simulink model "fluxrampdemodulationb"  (R2012b)
settings: Solver=ode45  StartTime=0.0  StopTime=10000  RelTol=1e-3
undefined symbols (not defined in the file): SL, transtable
libraries: xbsIndex_r4 x1338, casper_library_misc x8, xps_library x1
(part 1 of 13)
settings Model: Creator=tmadden  LastModifiedBy=tmadden

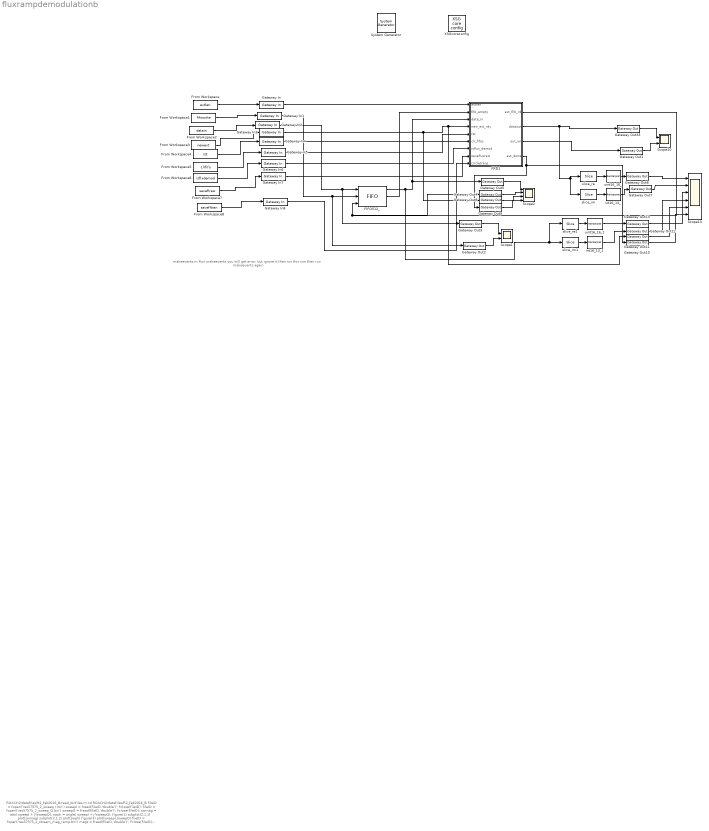
== system fluxrampdemodulationb ==
  note: makeevents.m
      | Run makeevents
      | you will get error, but ignore it
      | then run this sim
      | then run makeevents again
  note: ROACH2/datefiles/R2_feb2016_B/read_binfiles.m
      | cd ROACH2/datefiles/R2_feb2016_B
      |
      |
      |
      |
      |
      | fileID = fopen('res57575_2_sweep_I.bin')
      | sweepI = fread(fileID,'double')';
      | fclose(fileID);
      |
      |
      | fileID = fopen('res57575_2_sweep_Q.bin')
      | sweepQ = fread(fileID,'double')';
      | fclose(fileID);
      |
      |
      | swmag = abs( sweepI + j*sweepQ);
      |
      | swph = angle( sweepI + j*sweepQ);
      |
      | figure(1)
      | subplot(2,1,1)
      | plot(swmag)
      | subplot(2,1,2)
      | plot(swph)
      |
      | figure(3)
      | plot(sweepI,sweepQ)
      |
      |
      | fileID = fopen('res57575_2_stream_mag_ramp.bin')
      | mags = fread(fileID,'double')';
      | fclose(fileID);
      |
      |
      | fileID = fopen('res_57575_2_stream_phase_ramp.bin')
      | phasesr = fread(fileID,'double')';
      | fclose(fileID);
      |
      |
      |
      | nI = mags .* cos(phasesr);
      | nQ = mags .* sin(phasesr);
      |
      |
      | figure(3)
      | hold on
      | plot(nI,nQ,'r.')
      |
      |
      |
      |
      |
      | phases = phasesr / (pi);
      | phases = phases - 346;
      |
      |
      |
      | phases = [swph/pi , phases];
      | figure(4)
      | plot(phases(1:1000))
      |
      |
      | mags = [swmag , mags];
      |
      | magtime = timeseries(mags);
      | phasetime = timeseries(phases);
      |
      |
      | sync = zeros(1,length(phases));
      |
      | ping = 350;
      |
      | i = ping:100:length(phases);
      | sync(i) = 1;
      |
      |
      | synctime = timeseries(sync)
      |
      | figure(4)
      |
      | subplot(3,1,1)
      | plot(mags(1:400))
      | subplot(3,1,2)
      | plot(phases(1:400))
      | subplot(3,1,3)
      | plot(sync(1:400))
  " System Generator" : xbsIndex_r4/ System Generator  Tag=genX  xilinxfamily=Kintex7  part=xc7k325t  speed=-3  package=fbg676  synthesis_tool=XST  clock_wrapper=Clock Enables  directory=./netlist  proj_type=Project Navigator  Synth_file=XST Defaults  Impl_file=ISE Defaults  testbench=off  simulink_period=1  sysclk_period=10  dcm_input_clock_period=10  incr_netlist=off  trim_vbits=Everywhere in SubSystem  dbl_ovrd=According to Block Masks  core_generation=According to Block Masks  run_coregen=off  deprecated_control=off  eval_field=0  block_type=sysgen
  FIFO512_ : xbsIndex_r4/FIFO  mem_type=Block RAM  performance_options=First_Word_Fall_Through  infoedit1=Available only for V4, V5, V6, V7, K7, A7 and Zynq devices.  embedded_registers=off  depth=512  percent_nbits=1  rst=off  en=off  use_dcount=off  use_percent_full_port=off  use_almost_empty=off  almost_empty_thresh=2  use_almost_full=off  almost_full_thresh=256  dbl_ovrd=off  explicit_period=off  block_type=fifo
  FRD1 : Subsystem
  From Workspace : FromWorkspace  VariableName=evtlen  SampleTime=0  OutputAfterFinalValue=Holding final value
  From Workspace1 : FromWorkspace  VariableName=fifowrite  SampleTime=0  OutputAfterFinalValue=Holding final value
  From Workspace2 : FromWorkspace  VariableName=datain  Interpolate=off  OutputAfterFinalValue=Holding final value
  From Workspace3 : FromWorkspace  VariableName=newevt  SampleTime=0  OutputAfterFinalValue=Holding final value
  From Workspace4 : FromWorkspace  VariableName=rst  SampleTime=0  OutputAfterFinalValue=Holding final value
  From Workspace5 : FromWorkspace  VariableName=clrfifo  SampleTime=0  OutputAfterFinalValue=Holding final value
  From Workspace6 : FromWorkspace  VariableName=isflxdemod  SampleTime=0  OutputAfterFinalValue=Holding final value
  From Workspace7 : FromWorkspace  VariableName=saveflraw  SampleTime=0  OutputAfterFinalValue=Holding final value
  From Workspace8 : FromWorkspace  VariableName=savefltran  SampleTime=0  OutputAfterFinalValue=Holding final value
  Gateway In : xbsIndex_r4/Gateway In  gui_display_data_type=Fixed-point  arith_type=Unsigned  n_bits=8  bin_pt=0  preci_type=Single  exp_width=8  frac_width=24  quantization="Round  (unbiased: +/- Inf)"  overflow=Saturate  period=1  dbl_ovrd=off  timing_constraint=None  locs_specified=off  LOCs={}  UseAsADC=off  ADCChannel='1'  inherit_from_input=off  hdl_port=on  block_type=gatewayin
  Gateway In{1,3..8} (7 alike) : xbsIndex_r4/Gateway In  gui_display_data_type=Boolean  arith_type=Boolean  n_bits=16  bin_pt=14  preci_type=Single  exp_width=8  frac_width=24  quantization="Round  (unbiased: +/- Inf)"  overflow=Saturate  period=1  dbl_ovrd=off  timing_constraint=None  locs_specified=off  LOCs={}  UseAsADC=off  ADCChannel='1'  inherit_from_input=off  hdl_port=on  block_type=gatewayin
  Gateway In2 : xbsIndex_r4/Gateway In  gui_display_data_type=Fixed-point  arith_type=Unsigned  n_bits=32  bin_pt=0  preci_type=Single  exp_width=8  frac_width=24  quantization="Round  (unbiased: +/- Inf)"  overflow=Saturate  period=1  dbl_ovrd=off  timing_constraint=None  locs_specified=off  LOCs={}  UseAsADC=off  ADCChannel='1'  inherit_from_input=off  hdl_port=on  block_type=gatewayin
  Gateway Out{1..13,33} (14 alike) : xbsIndex_r4/Gateway Out  inherit_from_input=off  hdl_port=on  timing_constraint=None  locs_specified=off  LOCs={}  UseAsDAC=off  DACChannel='1'  block_type=gatewayout
  Scope1 : Scope  NumInputPorts=2
      settings: YMin=-5~-5  YMax=5~5  SaveName=output1  MaxDataPoints=1800
  Scope10 : Scope  NumInputPorts=2
      settings: YMin=-5~-5  YMax=5~5  SaveName=output  MaxDataPoints=1800
  Scope13 : Scope  NumInputPorts=6
      settings: YMin=-5~-5~-5~-5~-5~-5  YMax=5~5~5~5~5~5  SaveName=output3  MaxDataPoints=1800
  Scope2 : Scope  NumInputPorts=4
      settings: YMin=-5~-5~-5~-5  YMax=5~5~5~5  SaveName=output2  MaxDataPoints=1800
  XSGcoreconfig : xps_library/XSG core config  Tag=xps:xsg  hw_sys=ROACH2:sx475t  clk_src=sys_clk  ROACH_clk_src=sys_clk  ROACH2_clk_src=sys_clk  MKDIG_clk_src=sys_clk  clk_rate=128  sample_period=1  synthesis_tool=XST
  int16_13_ : xbsIndex_r4/Reinterpret  force_arith_type=on  arith_type="Signed  (2's comp)"  force_bin_pt=on  bin_pt=13  block_type=reinterpret
      settings: block_version=9.1.01
  int16_13_1 : xbsIndex_r4/Reinterpret  force_arith_type=on  arith_type="Signed  (2's comp)"  force_bin_pt=on  bin_pt=13  block_type=reinterpret
      settings: block_version=9.1.01
  slice_im : xbsIndex_r4/Slice  nbits=16  boolean_output=off  mode=Lower Bit Location + Width  bit1=0  base1=MSB of Input  bit0=0  base0=LSB of Input  dbl_ovrd=off  block_type=slice
      settings: block_version=9.1.01
  slice_im1 : xbsIndex_r4/Slice  nbits=16  boolean_output=off  mode=Lower Bit Location + Width  bit1=0  base1=MSB of Input  bit0=0  base0=LSB of Input  dbl_ovrd=off  block_type=slice
      settings: block_version=9.1.01
  slice_re : xbsIndex_r4/Slice  nbits=16  boolean_output=off  mode=Upper Bit Location + Width  bit1=0  base1=MSB of Input  bit0=0  base0=LSB of Input  dbl_ovrd=off  block_type=slice
      settings: block_version=9.1.01
  slice_re1 : xbsIndex_r4/Slice  nbits=16  boolean_output=off  mode=Upper Bit Location + Width  bit1=0  base1=MSB of Input  bit0=0  base0=LSB of Input  dbl_ovrd=off  block_type=slice
      settings: block_version=9.1.01
  uint16_16_ : xbsIndex_r4/Reinterpret  force_arith_type=on  arith_type=Unsigned  force_bin_pt=on  bin_pt=16  block_type=reinterpret
      settings: block_version=9.1.01
  uint16_16_1 : xbsIndex_r4/Reinterpret  force_arith_type=on  arith_type=Unsigned  force_bin_pt=on  bin_pt=16  block_type=reinterpret
      settings: block_version=9.1.01
  wires:
  Gateway In/1 -> FRD1/1(evtlen)
  Gateway In4/1 -> FRD1/5(rst)
  Gateway In5/1 -> FRD1/6(clr_fifos)
  Gateway In6/1 -> FRD1/7(isflux_demod)
  Gateway In7/1 -> FRD1/8(savefluxraw)
  From Workspace/1 -> Gateway In/1
  From Workspace1/1 -> Gateway In1/1
  From Workspace2/1 -> Gateway In2/1
  From Workspace3/1 -> Gateway In3/1
  From Workspace4/1 -> Gateway In4/1
  From Workspace5/1 -> Gateway In5/1
  From Workspace6/1 -> Gateway In6/1
  From Workspace7/1 -> Gateway In7/1
  Gateway Out33/1 -> Scope10/1
  FRD1/2(dataout) -> slice_im/1, slice_re/1, Gateway Out33/1
  Gateway Out1/1 -> Scope10/2
  FRD1/3(out_wr) -> Gateway Out1/1
  Gateway Out3/1 -> Scope1/1
  Gateway Out2/1 -> Scope1/2
  Gateway In3/1 -> Gateway Out8/1, FRD1/4(new_evt_rdy), Gateway Out11/1
  Gateway In2/1 -> Gateway Out3/1, FIFO512_/1
  FIFO512_/1 -> slice_re1/1, slice_im1/1, FRD1/3(data_in), Gateway Out5/1
  FRD1/1(evt_fifo_rd) -> FIFO512_/3, Gateway Out4/1
  FIFO512_/2 -> FRD1/2(fifo_empty)
  Gateway In1/1 -> Gateway Out2/1, FIFO512_/2
  Gateway Out5/1 -> Scope2/1
  Gateway Out4/1 -> Scope2/2
  From Workspace8/1 -> Gateway In8/1
  Gateway In8/1 -> FRD1/9(circletrans)
  slice_re/1 -> uint16_16_/1
  slice_im/1 -> int16_13_/1
  uint16_16_/1 -> Gateway Out6/1
  Gateway Out6/1 -> Scope13/1
  int16_13_/1 -> Gateway Out7/1
  Gateway Out7/1 -> Scope13/2
  Gateway Out8/1 -> Scope2/3
  Gateway Out9/1 -> Scope2/4
  FRD1/4(evt_done) -> Gateway Out10/1, Gateway Out9/1
  slice_re1/1 -> uint16_16_1/1
  slice_im1/1 -> int16_13_1/1
  uint16_16_1/1 -> Gateway Out13/1
  int16_13_1/1 -> Gateway Out12/1
  Gateway Out13/1 -> Scope13/3
  Gateway Out12/1 -> Scope13/4
  Gateway Out11/1 -> Scope13/5
  Gateway Out10/1 -> Scope13/6

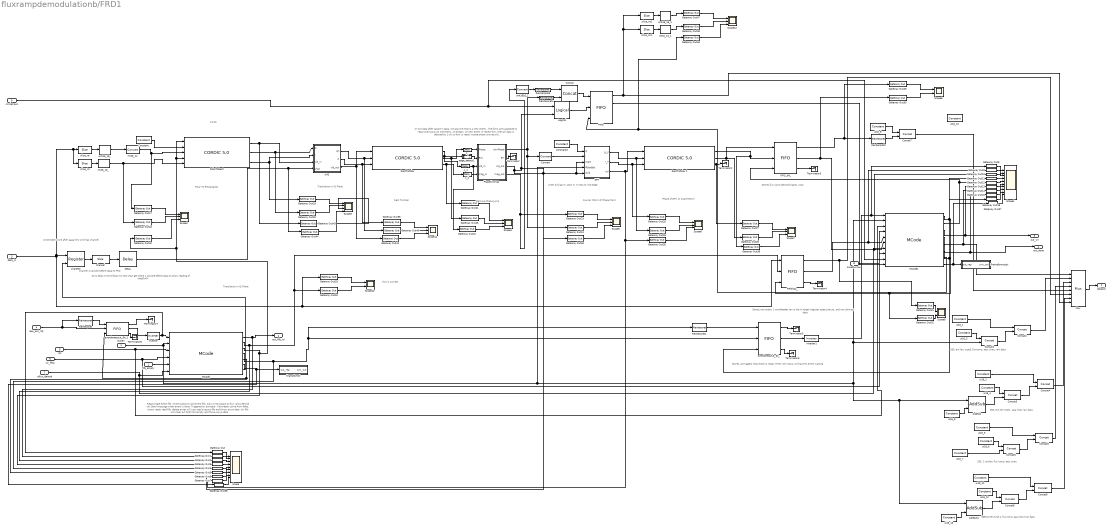
== system fluxrampdemodulationb/FRD1 ==
  note: stroe 32bit word after aaaa
      | this wird has channel
  note: 20 is delay time of polar to rect
      | chan get there 1 sample before data
      | to allow reading of theBRAM
  note: channel 1 sample before
      | data to FRD
  note: Z=20
  note: on 1st data after pause in data, we assume that is a new event...
      | the fsms are supposed to read continuous on one event...no breaks.
      | on new event, it resets fsm. then all data is delayed bu 1 clk so fsm
      | is ready insode phase unwrap ckt.
  note: this is correct
  note: 555, evt len type1 , aaa chan raw data
  note: 555, evt len, type3, fluxramp, aaa, chan, raw data
  note: 555, 2, evtlen, flux ramp, aaa, chan,
  note: Stores flux ramp dempd [hases. chan
  note: when dvld go hi, start it. it resp to rise edge
  note: Polar To Rectangular
  note: Translation in IQ Plane
  note: Remove Phase Jump
  note: Fourier Xform
      | Of Phase Term
  note: Rect To Polar
  note: Phase of DFT,
      | or Atan(Re/Im)
  note: Translation in IQ Plane
  note: Stores raw event.
      | 2 wordheader
      | len is the in length register
      | aaaa,chan,ts, and raw ph/mag data
  note: Stores up triggers that event is ready
      | When not mptuy we have en event waiting
  note: Read single event fifo.
      | Write output to 2nd event fifo.
      | Also write output to flux ramp demod ckt
      | Send message when event is done.
      | Triggered by evtready. if evtready come from fofop, clrevt ready read fifo.
      | delete evnet will just read sing evt fifo and throw awya data.
      | ckr fifo will clear evt fuifo intil empty and throw awya data
  note: 5555,evlen,type 4, fluxramp, aaa chan tran data
  evtlen : Inport
  fifo_empty : Inport  Port=2
  data_in : Inport  Port=3
  new_evt_rdy : Inport  Port=4
  rst : Inport  Port=5
  clr_fifos : Inport  Port=6
  isflux_demod : Inport  Port=7
  savefluxraw : Inport  Port=8
  circletrans : Inport  Port=9
  AddSub : xbsIndex_r4/AddSub  mode=Addition  use_carryin=off  use_carryout=off  en=off  latency=1  precision=User Defined  arith_type=Unsigned  n_bits=8  bin_pt=0  quantization=Truncate  overflow=Wrap  dbl_ovrd=off  use_behavioral_HDL=off  hw_selection=Fabric  pipelined=off  block_type=addsub
  AddSub1 : xbsIndex_r4/AddSub  mode=Addition  use_carryin=off  use_carryout=off  en=off  latency=1  precision=User Defined  arith_type=Unsigned  n_bits=8  bin_pt=0  quantization=Truncate  overflow=Wrap  dbl_ovrd=off  use_behavioral_HDL=off  hw_selection=Fabric  pipelined=off  block_type=addsub
  Concat{,1..9} (10 alike) : xbsIndex_r4/Concat  num_inputs=2  dbl_ovrd=off  block_type=concat
  Constant : xbsIndex_r4/Constant  const=0  gui_display_data_type=Fixed-point  arith_type=Signed (2's comp)  n_bits=16  bin_pt=14  preci_type=Single  exp_width=8  frac_width=24  explicit_period=on  period=1  equ=P=C  opselect=C  inp2=PCIN>>17  opr=+  inp1=P  carry=CIN  dbl_ovrd=off  block_type=constant
  Constant3 : xbsIndex_r4/Constant  const=0  gui_display_data_type=Fixed-point  arith_type=Signed (2's comp)  n_bits=16  bin_pt=14  preci_type=Single  exp_width=8  frac_width=24  explicit_period=on  period=1  equ=P=C  opselect=C  inp2=PCIN>>17  opr=+  inp1=P  carry=CIN  dbl_ovrd=off  block_type=constant
  Convert : xbsIndex_r4/Convert  gui_display_data_type=Fixed-point  arith_type="Signed  (2's comp)"  n_bits=16  bin_pt=14  float_type=Single  exp_bits=8  fraction_bits=24  quantization=Truncate  overflow=Wrap  en=off  latency=0  dbl_ovrd=off  pipeline=off  block_type=convert
  DFT : Subsystem
  Delay : xbsIndex_r4/Delay  rst=off  infoeditControl=Selection of Reset will increase slice count due to use of real FFs and instead of SRLs  en=off  latency=19  dbl_ovrd=off  reg_retiming=off  block_type=delay
  FIFO : xbsIndex_r4/FIFO  mem_type=Block RAM  performance_options=First_Word_Fall_Through  infoedit1=Available only for V4, V5, V6, V7, K7, A7 and Zynq devices.  embedded_registers=off  depth=512  percent_nbits=1  rst=off  en=off  use_dcount=off  use_percent_full_port=on  use_almost_empty=off  almost_empty_thresh=2  use_almost_full=off  almost_full_thresh=14  dbl_ovrd=off  explicit_period=off  block_type=fifo
  FIFO512_ : xbsIndex_r4/FIFO  mem_type=Block RAM  performance_options=First_Word_Fall_Through  infoedit1=Available only for V4, V5, V6, V7, K7, A7 and Zynq devices.  embedded_registers=off  depth=512  percent_nbits=1  rst=off  en=off  use_dcount=off  use_percent_full_port=off  use_almost_empty=off  almost_empty_thresh=2  use_almost_full=off  almost_full_thresh=256  dbl_ovrd=off  explicit_period=off  block_type=fifo
  FIFO_64_ : xbsIndex_r4/FIFO  mem_type=Block RAM  performance_options=First_Word_Fall_Through  infoedit1=Available only for V4, V5, V6, V7, K7, A7 and Zynq devices.  embedded_registers=off  depth=64  percent_nbits=1  rst=off  en=off  use_dcount=off  use_percent_full_port=off  use_almost_empty=off  almost_empty_thresh=2  use_almost_full=off  almost_full_thresh=32  dbl_ovrd=off  explicit_period=off  block_type=fifo
  Gateway Out{,1..49} (50 alike) : xbsIndex_r4/Gateway Out  inherit_from_input=off  hdl_port=on  timing_constraint=None  locs_specified=off  LOCs={}  UseAsDAC=off  DACChannel='1'  block_type=gatewayout
  Inverter : xbsIndex_r4/Inverter  en=off  latency=0  dbl_ovrd=off  block_type=inv
  Inverter1 : xbsIndex_r4/Inverter  en=off  latency=0  dbl_ovrd=off  block_type=inv
  Logical : xbsIndex_r4/Logical  logical_function=AND  inputs=2  en=off  latency=0  precision=Full  arith_type=Unsigned  n_bits=16  bin_pt=0  align_bp=on  dbl_ovrd=off  block_type=logical
  MCode : xbsIndex_r4/MCode  mfname=fluxRampFSM.m  explicit_period=off  period=1  inputsTable={'boundInpExpr'=>['','','','','',''],'inputs'=>['event_rdy','event_length','rst','clr_fifos','fifo_empty','is_fluxrampdemod']}  outputsTable={'outputs'=>['eventfifo_rd','outfifo_wr','demod_wr','event_done','clr_evt_rdy','stout'],'suppressOut'=>['off','off','off','off','off','off']}  dbl_ovrd=off  enable_stdout=off  enable_debug=off  suppress_output=on  defparams={}  hide_port_list={}  block_type=mcode
  MCode1 : xbsIndex_r4/MCode  mfname=fluxRampFSMOut2  explicit_period=on  period=1  inputsTable={'boundInpExpr'=>['','','','','','','',''],'inputs'=>['event_rdy','event_length','rst','clr_fifos','rawevt_fifo_empty','fluxrmp_fifo_empy','is_fluxrampdemod','is_savefluxraw']}  outputsTable={'outputs'=>['eventfifo_rd','fluxfifo_rd','outfifo_wr','wr_select','event_done','clr_evt_rdy','stout'],'suppressOut'=>['off','off','off','off','off','off','off']}  dbl_ovrd=off  enable_stdout=off  enable_debug=off  suppress_output=on  defparams={}  hide_port_list={}  block_type=mcode
  Mux : xbsIndex_r4/Mux  inputs=7  en=off  latency=0  precision=Full  arith_type=Unsigned  n_bits=16  bin_pt=14  quantization=Truncate  overflow=Wrap  dbl_ovrd=off  block_type=mux
  PhaseUnwrap : Subsystem
  "PolarToRect " : xbsIndex_r4/CORDIC 5.0   functional_selection=Rotate  architectural_configuration=Parallel  pipelining_mode=Maximum  data_format=SignedFraction  phase_format=Scaled_Radians  input_width=16  output_width=16  round_mode=Truncate  iterations=0  precision=0  compensation_scaling=Embedded_Multiplier  coarse_rotation=on  aclken=off  aresetn=off  out_tready=off  cartesian_has_tuser=off  cartesian_has_tlast=off  cartesian_tuser_width=1  phase_has_tuser=off  phase_has_tlast=off  phase_tuser_width=1  out_tlast_behv=Null  flow_control=NonBlocking  optimize_goal=Performance  trim_axipin_name=on  ip_name=CORDIC  ip_version=5.0  dsptool_ready=true  ipcore_usecache=true  ipcore_useipmodelcache=true  wrapper_available=true  port_translation_map={ 'aclken' => 'en', 'aresetn' => 'rst' }  block_type=cordic_v5_0
      settings: infoedit=CORDIC 5.0
  "RectToPolar " : xbsIndex_r4/CORDIC 5.0   functional_selection=Translate  architectural_configuration=Parallel  pipelining_mode=Maximum  data_format=SignedFraction  phase_format=Scaled_Radians  input_width=16  output_width=16  round_mode=Truncate  iterations=0  precision=0  compensation_scaling=Embedded_Multiplier  coarse_rotation=on  aclken=off  aresetn=off  out_tready=off  cartesian_has_tuser=off  cartesian_has_tlast=off  cartesian_tuser_width=1  phase_has_tuser=off  phase_has_tlast=off  phase_tuser_width=1  out_tlast_behv=Null  flow_control=NonBlocking  optimize_goal=Performance  trim_axipin_name=on  ip_name=CORDIC  ip_version=5.0  dsptool_ready=true  ipcore_usecache=true  ipcore_useipmodelcache=true  wrapper_available=true  port_translation_map={ 'aclken' => 'en', 'aresetn' => 'rst' }  block_type=cordic_v5_0
      settings: infoedit=CORDIC 5.0
  RectToPolar 1 : xbsIndex_r4/CORDIC 5.0   functional_selection=Translate  architectural_configuration=Parallel  pipelining_mode=Maximum  data_format=SignedFraction  phase_format=Scaled_Radians  input_width=16  output_width=16  round_mode=Truncate  iterations=0  precision=0  compensation_scaling=Embedded_Multiplier  coarse_rotation=on  aclken=off  aresetn=off  out_tready=off  cartesian_has_tuser=off  cartesian_has_tlast=off  cartesian_tuser_width=1  phase_has_tuser=off  phase_has_tlast=off  phase_tuser_width=1  out_tlast_behv=Null  flow_control=NonBlocking  optimize_goal=Performance  trim_axipin_name=on  ip_name=CORDIC  ip_version=5.0  dsptool_ready=true  ipcore_usecache=true  ipcore_useipmodelcache=true  wrapper_available=true  port_translation_map={ 'aclken' => 'en', 'aresetn' => 'rst' }  block_type=cordic_v5_0
      settings: infoedit=CORDIC 5.0
  Reinterpret : xbsIndex_r4/Reinterpret  force_arith_type=on  arith_type=Unsigned  force_bin_pt=off  bin_pt=0  block_type=reinterpret
  Reinterpret1 : xbsIndex_r4/Reinterpret  force_arith_type=on  arith_type=Unsigned  force_bin_pt=off  bin_pt=0  block_type=reinterpret
  Reinterpret2 : xbsIndex_r4/Reinterpret  force_arith_type=on  arith_type=Unsigned  force_bin_pt=on  bin_pt=0  block_type=reinterpret
  Reinterpret3 : xbsIndex_r4/Reinterpret  force_arith_type=on  arith_type=Unsigned  force_bin_pt=on  bin_pt=0  block_type=reinterpret
  Reinterpret4 : xbsIndex_r4/Reinterpret  force_arith_type=on  arith_type=Unsigned  force_bin_pt=on  bin_pt=0  block_type=reinterpret
  Scope : Scope  NumInputPorts=9
      settings: YMin=-5~-5~-5~-5~-5~-5~-5~-5~-5  YMax=5~5~5~5~5~5~5~5~5  SaveName=boolscope2
  Scope1 : Scope  NumInputPorts=10
      settings: YMin=-5~-5~-5~-5~-5~-5~-5~-5~-5~-5  YMax=5~5~5~5~5~5~5~5~5~5  SaveName=boolscope3
  Scope10 : Scope  NumInputPorts=2
      settings: YMin=-5~-5  YMax=5~5  SaveName=outfsm2  MaxDataPoints=1800
  Scope{2,4..7,11..12} (7 alike) : Scope  NumInputPorts=3
      Scope11 settings: TimeRange=1240.478781284003  YMin=-5~-5~-5  YMax=5~5~5  SaveName=scope_aftertr  MaxDataPoints=1800
      Scope12 settings: YMin=-5~-5~-5  YMax=5~5~5  SaveName=ScopeData18  MaxDataPoints=1800
      Scope2 settings: YMin=-5~-5~-5  YMax=5~5~5  MaxDataPoints=1800
      Scope4 settings: YMin=-5~-5~-5  YMax=5~5~5  SaveName=ScopeData3  MaxDataPoints=1800
      Scope5 settings: YMin=-5~-5~-5  YMax=5~5~5  SaveName=ScopeData4  MaxDataPoints=1800
      Scope6 settings: YMin=-5~-5~-5  YMax=5~5~5  SaveName=ScopeData6  MaxDataPoints=1800
      Scope7 settings: YMin=-5~-5~-5  YMax=5~5~5  SaveName=outdftdata  MaxDataPoints=1800
  Scope3 : Scope  NumInputPorts=4
      settings: TimeRange=1240.478781284003  YMin=-5~-5~-5~-5  YMax=5~5~5~5  SaveName=scope_beforetr  MaxDataPoints=1800
  Scope8 : Scope  NumInputPorts=2
      settings: YMin=-5~-5  YMax=5~5  SaveName=ScopeData15  MaxDataPoints=1800
  Scope9 : Scope  NumInputPorts=2
      settings: YMin=-5~-5  YMax=5~5  SaveName=ScopeData16  MaxDataPoints=1800
  Terminator{,2..8} (8 alike) : Terminator
  chanReg : xbsIndex_r4/Register  init=0  rst=off  en=on  dbl_ovrd=off  block_type=register
  channel : xbsIndex_r4/Slice  nbits=8  boolean_output=off  mode=Lower Bit Location + Width  bit1=0  base1=MSB of Input  bit0=0  base0=LSB of Input  dbl_ovrd=off  block_type=slice
  edge_detect1 : Subsystem  AncestorBlock=casper_library_misc/edge_detect  mask(edge_detect){edge=Rising, polarity=Active High, x_in=[0 0.08 0.08 0.16 0.16 0.24 0.24 0.32 0.32 0.4], y_in=[-1 -1  1  1  1  1  1  1  1  1], x_out=[0.6 0.68 0.68 0.76 0.76 0.84 0.84 0.92 0.92 1], y_out=[-1 -1  1  1 -1 -1 -1 -1 -1 -1]}
      mask prompts: edge "Edge Type"; polarity "Output Polarity"; x_in "Input X Positions"; y_in "Input Y Positions"; x_out "Output X Positions"; y_out "Output Y Positions"
      mask help: Output is active for one-cycle after each edge of the specified type (i.e. rising, falling or both).
      mask init:
      | edge_detect_init(gcb,...
      |     'edge',edge,...
      |     'polarity',polarity,...
      |     'x_in',x_in,...
      |     'x_out',x_out,...
      |     'y_in',y_in,...
      |     'y_out',y_out);
      | 
      | x_in_num=str2num(getfield(getfield(get_param(gcb,'UserData'),'parameters'),'x_in'));
      | x_out_num=str2num(getfield(getfield(get_param(gcb,'UserData'),'parameters'),'x_out'));
      | y_in_num=str2num(getfield(getfield(get_param(gcb,'UserData'),'parameters'),'y_in'));
      | y_out_num=str2num(getfield(getfield(get_param(gcb,'UserData'),'parameters'),'y_out'));
      settings: AttributesFormatString=|
      | rising edges
      | active high
      mask Help: Output is active for one-cycle after each edge of the specified type (i.e. rising, falling, or both).  Latency is zero.
      mask TypeOptions edge: Rising | Falling | Both
      mask TypeOptions polarity: Active High | Active Low
      mask Display:
      | plot(x_in_num,0.5+y_in_num*0.2);
      | plot(x_out_num,0.5+y_out_num*0.2);
  evendonequtut_64_ : xbsIndex_r4/FIFO  mem_type=Block RAM  performance_options=First_Word_Fall_Through  infoedit1=Available only for V4, V5, V6, V7, K7, A7 and Zynq devices.  embedded_registers=off  depth=16  percent_nbits=1  rst=off  en=off  use_dcount=off  use_percent_full_port=off  use_almost_empty=off  almost_empty_thresh=2  use_almost_full=off  almost_full_thresh=14  dbl_ovrd=off  explicit_period=off  block_type=fifo
  evendonequtut_64_1 : xbsIndex_r4/FIFO  mem_type=Block RAM  performance_options=First_Word_Fall_Through  infoedit1=Available only for V4, V5, V6, V7, K7, A7 and Zynq devices.  embedded_registers=off  depth=16  percent_nbits=1  rst=off  en=off  use_dcount=off  use_percent_full_port=off  use_almost_empty=off  almost_empty_thresh=2  use_almost_full=off  almost_full_thresh=14  dbl_ovrd=off  explicit_period=off  block_type=fifo
  flrampfsmoutst : Subsystem  Tag=xps:sw_reg  AncestorBlock=xps_library/software register  mask(swreg){mode=one value, io_dir=To Processor, io_delay=0, sample_period=1, names=reg, bitwidths=5, arith_types=0, bin_pts=0, sim_port=on, show_format=off}
      mask prompts: io_dir "I/O direction"; io_delay "I/O delay"; sample_period "Sample period"; names "Name:"; bitwidths "Bitwidth:"; arith_types "Type (ufix=0, fix=1, bool=2):"; bin_pts "Binary pt:"; sim_port "Provide sim input/output?"; show_format "Print format string?"
      mask init:
      | swreg_init(gcb)
      settings: AttributesFormatString=1output
      mask TypeOptions mode: one value | fields of equal size | fields of arbitrary size
      mask Callback mode: swreg_cb(gcb);
      mask TypeOptions io_dir: To Processor | From Processor
      mask Callback io_dir:
      | mask_enables = get_param(gcb, 'MaskEnables');
      | mask_names = get_param(gcb, 'MaskNames');
      | if strcmp(get_param(gcb, 'io_dir'), 'To Processor'),
      |     mask_enables{ismember(mask_names, 'sample_period')} = 'off';
      | else
      |     mask_enables{ismember(mask_names, 'sample_period')} = 'on';
      | end
      | set_param(gcb, 'MaskEnables', mask_enables);
      mask Callback bitwidths:
      | swreg_maskcheck(gcb);
      | % blk = gcb;
      | % mode = get_param(blk, 'mode');
      | % current_widths = eval(get_param(blk, 'bitwidths'));
      | % if (strcmp(mode, 'one value') || strcmp(mode, 'fields of equal size')) && (length(current_widths) > 1),
      | %     error('Only one width may be specified for this mode.');
      | % elseif strcmp(mode, 'fields of arbitrary size')
      | %     current_names = textscan(strtrim(strrep(strrep(get_param(blk, 'names'), ']', ''), '[', '')), '%s');
      | %     current_names = current_names{1};
      | %     numios = length(current_names);
      | %     if length(current_widths) ~= numios,
      | %         error('%d field names specified, but %d widths?', numios, length(current_widths));
      | %     end
      | % end
      | % total_width = 0;
      | % for ctr = 1 : length(current_widths),
      | %     total_width = total_width + current_widths(ctr);
      | % end
      | % if total_width > 32,
      | %     error('Total width must be 32 or less, set to %d.', total_width);
      | % end
      mask Callback arith_types:
      | [numios, ~, ~, ~, current_types] = swreg_maskcheck(gcb);
      | % blk = gcb;
      | % mode = get_param(blk, 'mode');
      | % current_types = eval(get_param(blk, 'arith_types'));
      | % numios = length(current_types);
      | % if (strcmp(mode, 'one value') || strcmp(mode, 'fields of equal size')) && (length(current_types) > 1),
      | %     error('Only one type may be specified for this mode.');
      | % elseif strcmp(mode, 'fields of arbitrary size')
      | %     current_names = textscan(strtrim(strrep(strrep(get_param(blk, 'names'), ']', ''), '[', '')), '%s');
      | %     current_names = current_names{1};
      | %     numios = length(current_names);
      | %     if length(current_types) ~= numios,
      | %         error('%d field names specified, but %d types?', numios, length(current_types));
      | %     end
      | % end
      | problem = 0;
      | for ctr = 1 : numios,
      |     t = current_types(ctr);
      |     if (t < 0) || (t > 2),
      |         problem = t;
      |         ctr = numios + 1;
      |     end
      | end
      | if problem ~= 0,
      |     error('Type cannot be %i, must be 0, 1 or 2.', problem);
      | end
      mask Callback bin_pts:
      | swreg_maskcheck(gcb);
      | % blk = gcb;
      | % mode = get_param(blk, 'mode');
      | % current_bins = eval(get_param(blk, 'bin_pts'));
      | % if (strcmp(mode, 'one value') || strcmp(mode, 'fields of equal size')) && (length(current_bins) > 1),
      | %     error('Only one binary pt may be specified for this mode.');
      | % elseif strcmp(mode, 'fields of arbitrary size')
      | %     current_names = textscan(strtrim(strrep(strrep(get_param(blk, 'names'), ']', ''), '[', '')), '%s');
      | %     current_names = current_names{1};
      | %     numios = length(current_names);
      | %     if length(current_bins) ~= numios,
      | %         error('%d field names specified, but %d binary pts?', numios, length(current_bins));
      | %     end
      | % end
  flrampfsmst : Subsystem  Tag=xps:sw_reg  AncestorBlock=xps_library/software register  mask(swreg){mode=one value, io_dir=To Processor, io_delay=0, sample_period=1, names=reg, bitwidths=4, arith_types=0, bin_pts=0, sim_port=on, show_format=off}
      mask prompts: io_dir "I/O direction"; io_delay "I/O delay"; sample_period "Sample period"; names "Name:"; bitwidths "Bitwidth:"; arith_types "Type (ufix=0, fix=1, bool=2):"; bin_pts "Binary pt:"; sim_port "Provide sim input/output?"; show_format "Print format string?"
      mask init:
      | swreg_init(gcb)
      settings: AttributesFormatString=1output
      mask TypeOptions mode: one value | fields of equal size | fields of arbitrary size
      mask Callback mode: swreg_cb(gcb);
      mask TypeOptions io_dir: To Processor | From Processor
      mask Callback io_dir:
      | mask_enables = get_param(gcb, 'MaskEnables');
      | mask_names = get_param(gcb, 'MaskNames');
      | if strcmp(get_param(gcb, 'io_dir'), 'To Processor'),
      |     mask_enables{ismember(mask_names, 'sample_period')} = 'off';
      | else
      |     mask_enables{ismember(mask_names, 'sample_period')} = 'on';
      | end
      | set_param(gcb, 'MaskEnables', mask_enables);
      mask Callback bitwidths:
      | swreg_maskcheck(gcb);
      | % blk = gcb;
      | % mode = get_param(blk, 'mode');
      | % current_widths = eval(get_param(blk, 'bitwidths'));
      | % if (strcmp(mode, 'one value') || strcmp(mode, 'fields of equal size')) && (length(current_widths) > 1),
      | %     error('Only one width may be specified for this mode.');
      | % elseif strcmp(mode, 'fields of arbitrary size')
      | %     current_names = textscan(strtrim(strrep(strrep(get_param(blk, 'names'), ']', ''), '[', '')), '%s');
      | %     current_names = current_names{1};
      | %     numios = length(current_names);
      | %     if length(current_widths) ~= numios,
      | %         error('%d field names specified, but %d widths?', numios, length(current_widths));
      | %     end
      | % end
      | % total_width = 0;
      | % for ctr = 1 : length(current_widths),
      | %     total_width = total_width + current_widths(ctr);
      | % end
      | % if total_width > 32,
      | %     error('Total width must be 32 or less, set to %d.', total_width);
      | % end
      mask Callback arith_types:
      | [numios, ~, ~, ~, current_types] = swreg_maskcheck(gcb);
      | % blk = gcb;
      | % mode = get_param(blk, 'mode');
      | % current_types = eval(get_param(blk, 'arith_types'));
      | % numios = length(current_types);
      | % if (strcmp(mode, 'one value') || strcmp(mode, 'fields of equal size')) && (length(current_types) > 1),
      | %     error('Only one type may be specified for this mode.');
      | % elseif strcmp(mode, 'fields of arbitrary size')
      | %     current_names = textscan(strtrim(strrep(strrep(get_param(blk, 'names'), ']', ''), '[', '')), '%s');
      | %     current_names = current_names{1};
      | %     numios = length(current_names);
      | %     if length(current_types) ~= numios,
      | %         error('%d field names specified, but %d types?', numios, length(current_types));
      | %     end
      | % end
      | problem = 0;
      | for ctr = 1 : numios,
      |     t = current_types(ctr);
      |     if (t < 0) || (t > 2),
      |         problem = t;
      |         ctr = numios + 1;
      |     end
      | end
      | if problem ~= 0,
      |     error('Type cannot be %i, must be 0, 1 or 2.', problem);
      | end
      mask Callback bin_pts:
      | swreg_maskcheck(gcb);
      | % blk = gcb;
      | % mode = get_param(blk, 'mode');
      | % current_bins = eval(get_param(blk, 'bin_pts'));
      | % if (strcmp(mode, 'one value') || strcmp(mode, 'fields of equal size')) && (length(current_bins) > 1),
      | %     error('Only one binary pt may be specified for this mode.');
      | % elseif strcmp(mode, 'fields of arbitrary size')
      | %     current_names = textscan(strtrim(strrep(strrep(get_param(blk, 'names'), ']', ''), '[', '')), '%s');
      | %     current_names = current_names{1};
      | %     numios = length(current_names);
      | %     if length(current_bins) ~= numios,
      | %         error('%d field names specified, but %d binary pts?', numios, length(current_bins));
      | %     end
      | % end
  int16_13_ : xbsIndex_r4/Reinterpret  force_arith_type=on  arith_type="Signed  (2's comp)"  force_bin_pt=on  bin_pt=13  block_type=reinterpret
      settings: block_version=9.1.01
  int16_13_1 : xbsIndex_r4/Reinterpret  force_arith_type=on  arith_type="Signed  (2's comp)"  force_bin_pt=on  bin_pt=13  block_type=reinterpret
      settings: block_version=9.1.01
  int16_14 : xbsIndex_r4/Convert  gui_display_data_type=Fixed-point  arith_type="Signed  (2's comp)"  n_bits=16  bin_pt=14  float_type=Single  exp_bits=8  fraction_bits=24  quantization=Truncate  overflow=Wrap  en=off  latency=0  dbl_ovrd=off  pipeline=off  block_type=convert
  slice_im : xbsIndex_r4/Slice  nbits=16  boolean_output=off  mode=Lower Bit Location + Width  bit1=0  base1=MSB of Input  bit0=0  base0=LSB of Input  dbl_ovrd=off  block_type=slice
      settings: block_version=9.1.01
  slice_im1 : xbsIndex_r4/Slice  nbits=16  boolean_output=off  mode=Lower Bit Location + Width  bit1=0  base1=MSB of Input  bit0=0  base0=LSB of Input  dbl_ovrd=off  block_type=slice
      settings: block_version=9.1.01
  slice_re : xbsIndex_r4/Slice  nbits=16  boolean_output=off  mode=Upper Bit Location + Width  bit1=0  base1=MSB of Input  bit0=0  base0=LSB of Input  dbl_ovrd=off  block_type=slice
      settings: block_version=9.1.01
  slice_re1 : xbsIndex_r4/Slice  nbits=16  boolean_output=off  mode=Upper Bit Location + Width  bit1=0  base1=MSB of Input  bit0=0  base0=LSB of Input  dbl_ovrd=off  block_type=slice
      settings: block_version=9.1.01
  trIQ : Subsystem
  ui16_{1..2,5,10..11} (5 alike) : xbsIndex_r4/Constant  const=21845  gui_display_data_type=Fixed-point  arith_type=Unsigned  n_bits=16  bin_pt=0  preci_type=Single  exp_width=8  frac_width=24  explicit_period=on  period=1  equ=P=C  opselect=C  inp2=PCIN>>17  opr=+  inp1=P  carry=CIN  dbl_ovrd=off  block_type=constant
  ui16_12 : xbsIndex_r4/Constant  const=4  gui_display_data_type=Fixed-point  arith_type=Unsigned  n_bits=8  bin_pt=0  preci_type=Single  exp_width=8  frac_width=24  explicit_period=on  period=1  equ=P=C  opselect=C  inp2=PCIN>>17  opr=+  inp1=P  carry=CIN  dbl_ovrd=off  block_type=constant
  ui16_13 : xbsIndex_r4/Constant  const=2  gui_display_data_type=Fixed-point  arith_type=Unsigned  n_bits=8  bin_pt=0  preci_type=Single  exp_width=8  frac_width=24  explicit_period=on  period=1  equ=P=C  opselect=C  inp2=PCIN>>17  opr=+  inp1=P  carry=CIN  dbl_ovrd=off  block_type=constant
  ui16_3 : xbsIndex_r4/Constant  const=3  gui_display_data_type=Fixed-point  arith_type=Unsigned  n_bits=8  bin_pt=0  preci_type=Single  exp_width=8  frac_width=24  explicit_period=on  period=1  equ=P=C  opselect=C  inp2=PCIN>>17  opr=+  inp1=P  carry=CIN  dbl_ovrd=off  block_type=constant
  ui16_4 : xbsIndex_r4/Constant  const=1  gui_display_data_type=Fixed-point  arith_type=Unsigned  n_bits=8  bin_pt=0  preci_type=Single  exp_width=8  frac_width=24  explicit_period=on  period=1  equ=P=C  opselect=C  inp2=PCIN>>17  opr=+  inp1=P  carry=CIN  dbl_ovrd=off  block_type=constant
  ui16_6 : xbsIndex_r4/Constant  const=2  gui_display_data_type=Fixed-point  arith_type=Unsigned  n_bits=8  bin_pt=0  preci_type=Single  exp_width=8  frac_width=24  explicit_period=on  period=1  equ=P=C  opselect=C  inp2=PCIN>>17  opr=+  inp1=P  carry=CIN  dbl_ovrd=off  block_type=constant
  ui16_7 : xbsIndex_r4/Constant  const=3  gui_display_data_type=Fixed-point  arith_type=Unsigned  n_bits=8  bin_pt=0  preci_type=Single  exp_width=8  frac_width=24  explicit_period=on  period=1  equ=P=C  opselect=C  inp2=PCIN>>17  opr=+  inp1=P  carry=CIN  dbl_ovrd=off  block_type=constant
  ui16_8 : xbsIndex_r4/Constant  const=2  gui_display_data_type=Fixed-point  arith_type=Unsigned  n_bits=8  bin_pt=0  preci_type=Single  exp_width=8  frac_width=24  explicit_period=on  period=1  equ=P=C  opselect=C  inp2=PCIN>>17  opr=+  inp1=P  carry=CIN  dbl_ovrd=off  block_type=constant
  ui16_9 : xbsIndex_r4/Constant  const=0  gui_display_data_type=Fixed-point  arith_type=Unsigned  n_bits=16  bin_pt=0  preci_type=Single  exp_width=8  frac_width=24  explicit_period=on  period=1  equ=P=C  opselect=C  inp2=PCIN>>17  opr=+  inp1=P  carry=CIN  dbl_ovrd=off  block_type=constant
  uint1616_1 : xbsIndex_r4/Convert  gui_display_data_type=Fixed-point  arith_type=Unsigned  n_bits=16  bin_pt=16  float_type=Single  exp_bits=8  fraction_bits=24  quantization=Truncate  overflow=Wrap  en=off  latency=0  dbl_ovrd=off  pipeline=off  block_type=convert
  uint16_16_ : xbsIndex_r4/Reinterpret  force_arith_type=on  arith_type=Unsigned  force_bin_pt=on  bin_pt=16  block_type=reinterpret
      settings: block_version=9.1.01
  uint16_16_1 : xbsIndex_r4/Reinterpret  force_arith_type=on  arith_type=Unsigned  force_bin_pt=on  bin_pt=16  block_type=reinterpret
      settings: block_version=9.1.01
  z_ : xbsIndex_r4/Delay  rst=off  infoeditControl=Selection of Reset will increase slice count due to use of real FFs and instead of SRLs  en=off  latency=1  dbl_ovrd=off  reg_retiming=off  block_type=delay
  z_1 : xbsIndex_r4/Delay  rst=off  infoeditControl=Selection of Reset will increase slice count due to use of real FFs and instead of SRLs  en=off  latency=1  dbl_ovrd=off  reg_retiming=off  block_type=delay
  z_2 : xbsIndex_r4/Delay  rst=off  infoeditControl=Selection of Reset will increase slice count due to use of real FFs and instead of SRLs  en=off  latency=1  dbl_ovrd=off  reg_retiming=off  block_type=delay
  evt_fifo_rd : Outport
  dataout : Outport  Port=2
  out_wr : Outport  Port=3
  evt_done : Outport  Port=4
  wires:
  fifo_empty/1 -> MCode/5
  MCode/1 -> Gateway Out1/1, evt_fifo_rd/1
  edge_detect1/1(out) -> PhaseUnwrap/2(Rst)
  MCode/4 -> Gateway Out4/1, Reinterpret1/1, evendonequtut_64_/2
  "PolarToRect "/1 -> Gateway Out43/1, trIQ/3(vld_in)
  DFT/1(Q_F) -> Gateway Out26/1, RectToPolar 1/2
  MCode1/4 -> Gateway Out14/1, Mux/1
  uint16_16_/1 -> int16_14/1
  FIFO512_/3 -> Terminator4/1
  evendonequtut_64_/3 -> Terminator6/1
  trIQ/3(vld_out) -> Gateway Out41/1, "RectToPolar "/1
  evendonequtut_64_/1 -> Terminator5/1
  "RectToPolar "/1 -> z_1/1, edge_detect1/1(in)
  "PolarToRect "/2 -> Gateway Out20/1, trIQ/1(Q)
  MCode/5 -> Gateway Out5/1, evendonequtut_64_1/3
  "PolarToRect "/3 -> Gateway Out19/1, trIQ/2(I)
  "RectToPolar "/3 -> Gateway Out21/1, z_2/1
  trIQ/2(It) -> Gateway Out39/1, "RectToPolar "/3
  data_in/1 -> slice_im/1, slice_re/1, chanReg/1, Gateway Out33/1, FIFO512_/1
  DFT/3(vld) -> Gateway Out35/1, Gateway Out7/1, RectToPolar 1/1
  Constant/1 -> "PolarToRect "/2
  Constant3/1 -> DFT/1(Q)
  PhaseUnwrap/1(UwrPhase) -> Reinterpret4/1, Gateway Out24/1, Convert/1
  PhaseUnwrap/2(Err) -> Terminator/1
  FIFO_64_/2 -> Gateway Out30/1, Gateway Out10/1, MCode1/6
  rst/1 -> MCode1/3, MCode/3
  evendonequtut_64_1/3 -> Terminator8/1
  MCode1/3 -> Gateway Out13/1, out_wr/1
  Inverter1/1 -> Gateway Out8/1, MCode1/1
  DFT/2(I_F) -> Gateway Out25/1, RectToPolar 1/3
  FIFO512_/2 -> Gateway Out9/1, MCode1/5
  MCode1/6 -> evendonequtut_64_/3, Gateway Out16/1
  Inverter/1 -> Gateway Out/1, MCode/1
  MCode1/5 -> Gateway Out15/1, evt_done/1
  evendonequtut_64_/2 -> Inverter1/1
  evendonequtut_64_1/1 -> Terminator7/1
  RectToPolar 1/3 -> Gateway Out27/1, Terminator2/1
  evendonequtut_64_1/2 -> Inverter/1
  PhaseUnwrap/4(mag_out) -> uint1616_1/1, Gateway Out23/1
  int16_13_/1 -> Gateway Out18/1, "PolarToRect "/5
  clr_fifos/1 -> MCode/4, MCode1/4
  new_evt_rdy/1 -> Reinterpret/1, evendonequtut_64_1/2
  "RectToPolar "/2 -> Gateway Out45/1, z_/1
  FIFO_64_/3 -> Terminator3/1
  trIQ/1(Qt) -> Gateway Out40/1, "RectToPolar "/2
  MCode1/2 -> Gateway Out12/1, FIFO_64_/3
  MCode/2 -> Gateway Out2/1, Gateway Out34/1, FIFO512_/2
  MCode/3 -> Gateway Out3/1, "PolarToRect "/1, "PolarToRect "/4, Gateway Out42/1
  isflux_demod/1 -> MCode1/7, MCode/6
  ui16_1/1 -> Concat2/1
  Concat1/1 -> Concat2/2
  ui16_3/1 -> Concat1/1
  Concat2/1 -> Mux/2
  Concat7/1 -> Mux/5
  FIFO512_/1 -> Gateway Out31/1, Mux/6
  ui16_2/1 -> Concat4/1
  Concat3/1 -> Concat4/2
  ui16_4/1 -> Concat3/1
  ui16_5/1 -> Concat6/1
  Concat5/1 -> Concat6/2
  ui16_6/1 -> Concat5/1
  ui16_7/1 -> Concat5/2
  Concat4/1 -> Mux/3
  Concat6/1 -> Mux/4
  ui16_8/1 -> AddSub/2
  AddSub/1 -> Concat3/2
  savefluxraw/1 -> MCode1/8
  Reinterpret/1 -> evendonequtut_64_1/1
  Reinterpret1/1 -> evendonequtut_64_/1
  Gateway Out/1 -> Scope/1
  Gateway Out1/1 -> Scope/2
  Gateway Out2/1 -> Scope/3
  Gateway Out3/1 -> Scope/4
  Gateway Out4/1 -> Scope/5
  Gateway Out5/1 -> Scope/6
  Gateway Out6/1 -> Scope/7
  Gateway Out7/1 -> Scope/8
  RectToPolar 1/1 -> Gateway Out36/1, FIFO_64_/2
  Gateway Out8/1 -> Scope1/1
  Gateway Out9/1 -> Scope1/2
  Gateway Out10/1 -> Scope1/3
  Gateway Out11/1 -> Scope1/4
  Gateway Out12/1 -> Scope1/5
  Gateway Out13/1 -> Scope1/6
  Gateway Out14/1 -> Scope1/7
  Gateway Out15/1 -> Scope1/8
  Gateway Out16/1 -> Scope1/9
  Gateway Out18/1 -> Scope2/2
  Gateway Out17/1 -> Scope2/1
  Gateway Out20/1 -> Scope3/2
  Gateway Out19/1 -> Scope3/1
  Gateway Out21/1 -> Scope4/1
  Gateway Out24/1 -> Scope5/2
  Gateway Out23/1 -> Scope5/1
  Gateway Out26/1 -> Scope6/2
  Gateway Out25/1 -> Scope6/1
  Gateway Out28/1 -> Scope7/2
  Gateway Out27/1 -> Scope7/1
  RectToPolar 1/2 -> Gateway Out28/1, FIFO_64_/1
  Gateway Out30/1 -> Scope8/2
  Gateway Out29/1 -> Scope8/1
  Gateway Out32/1 -> Scope9/2
  Gateway Out31/1 -> Scope9/1
  MCode1/1 -> Gateway Out11/1, Gateway Out32/1, FIFO512_/3
  Mux/1 -> dataout/1
  Gateway Out34/1 -> Scope10/2
  Gateway Out33/1 -> Scope10/1
  Reinterpret2/1 -> Concat7/2
  FIFO_64_/1 -> Gateway Out29/1, Reinterpret2/1
  ui16_9/1 -> Concat7/1
  slice_re/1 -> uint16_16_/1
  slice_im/1 -> int16_13_/1
  int16_14/1 -> Gateway Out17/1, "PolarToRect "/3
  MCode1/7 -> Gateway Out37/1, flrampfsmoutst/1(out_reg)
  z_1/1 -> Gateway Out22/1, PhaseUnwrap/3(vld_in)
  z_2/1 -> PhaseUnwrap/4(mag_in)
  z_/1 -> PhaseUnwrap/1(Phase)
  Gateway Out35/1 -> Scope6/3
  Gateway Out36/1 -> Scope7/3
  Gateway Out37/1 -> Scope1/10
  Gateway Out38/1 -> Scope/9
  MCode/6 -> Gateway Out38/1, flrampfsmst/1(out_reg)
  Gateway Out40/1 -> Scope11/2
  Gateway Out39/1 -> Scope11/1
  Gateway Out41/1 -> Scope11/3
  Gateway Out42/1 -> Scope2/3
  Gateway Out43/1 -> Scope3/3
  MCode/7 -> chanReg/2
  chanReg/1 -> channel/1
  channel/1 -> Delay/1
  Delay/1 -> Gateway Out44/1, trIQ/4(chan)
  Gateway Out44/1 -> Scope3/4
  Concat/1 -> FIFO/1
  PhaseUnwrap/3(vld_out) -> Gateway Out46/1, Logical/2, DFT/3(start), DFT/5(dvld), Gateway Out6/1
  Logical/1 -> FIFO/2
  FIFO/2 -> MCode1/10
  circletrans/1 -> MCode1/9, Logical/1
  ui16_11/1 -> Concat9/1
  Concat8/1 -> Concat9/2
  ui16_12/1 -> Concat8/1
  evtlen/1 -> MCode/2, DFT/4(fftlen8bit), Concat1/2, MCode1/2, AddSub1/1, AddSub/1
  ui16_13/1 -> AddSub1/2
  AddSub1/1 -> Concat8/2
  Concat9/1 -> Mux/7
  FIFO/1 -> slice_im1/1, slice_re1/1, Mux/8
  MCode1/8 -> Gateway Out49/1, FIFO/3
  Reinterpret4/1 -> Concat/2
  Reinterpret3/1 -> Concat/1
  Gateway Out22/1 -> Scope4/3
  Gateway Out45/1 -> Scope4/2
  Gateway Out46/1 -> Scope5/3
  Gateway Out48/1 -> Scope12/2
  Gateway Out47/1 -> Scope12/1
  Gateway Out49/1 -> Scope12/3
  slice_re1/1 -> uint16_16_1/1
  slice_im1/1 -> int16_13_1/1
  uint16_16_1/1 -> Gateway Out47/1
  int16_13_1/1 -> Gateway Out48/1
  Convert/1 -> DFT/2(I)
  uint1616_1/1 -> Reinterpret3/1
